simulink model "CruiseControlWithPID"  (R2021b)
settings: Solver=VariableStepAuto  StartTime=0.0  StopTime=50  FixedStep=0.01  RelTol=1e-3
PreLoadFcn:
  | clear;
  | CC_PID
values from neighbouring files (symbols this model uses):
  CC_b_Cn = 50    [CC_PID.m]
  CC_m_Cn = 1000    [CC_PID.m]
settings Model: Creator=banashreen  LastModifiedBy=Dell-pc
settings SolverCC: AlgebraicLoopSolver=TrustRegion
settings DataIOCC: ReturnWorkspaceOutputs=off
settings DebuggingCC: SFMachineParentedDataDiag=warning  ArithmeticOperatorsInVariantConditions=warning
settings SFSimCC: SimUseLocalCustomCode=off  CustomCodeUndefinedFunction=UseInterfaceOnly
settings RTWCC: RTWUseLocalCustomCode=off
settings ConfigComp: CovScope=ReferencedModels  CovIncludeTopModel=off

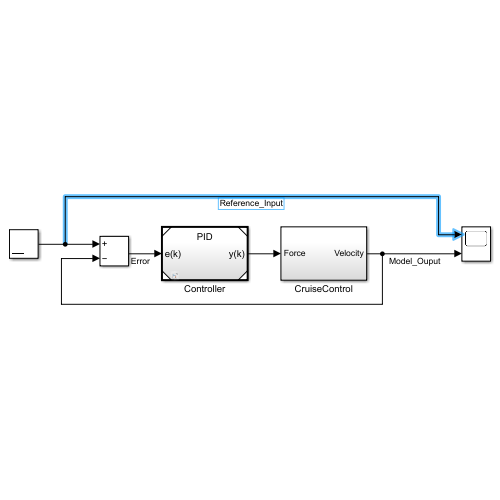
[thumbnail: Simulink's stored preview of the top-level diagram]
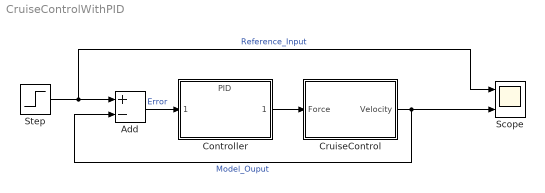
== system CruiseControlWithPID ==
  Add : Sum  Inputs=+-
  Controller : ModelReference  ModelNameDialog=PID.slx  SimulationMode=Normal  ShowModelTerminatePort=on  ModelReferenceVersion=9.3
  CruiseControl : Subsystem
  Scope : Scope  NumInputPorts=2
  Step : Step  Time=5  After=100  SampleTime=0
  wires:
  Step/1 -> Scope/1, Add/1  "Reference_Input"
  CruiseControl/1(Velocity) -> Add/2, Scope/2  "Model_Ouput"
  Controller/1 -> CruiseControl/1(Force)
  Add/1 -> Controller/1  "Error"

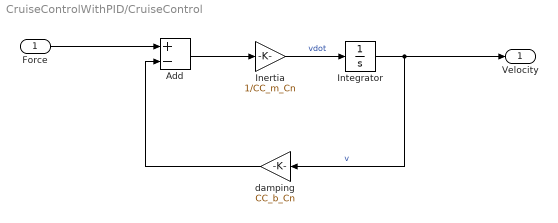
== system CruiseControlWithPID/CruiseControl ==
  Force : Inport
  Add : Sum  Inputs=+-
  Inertia : Gain  Gain=1/CC_m_Cn
  Integrator : Integrator
  damping : Gain  Gain=CC_b_Cn
  Velocity : Outport  VectorParamsAs1DForOutWhenUnconnected=off
  wires:
  Force/1 -> Add/1
  Add/1 -> Inertia/1
  Inertia/1 -> Integrator/1  "vdot"
  damping/1 -> Add/2
  Integrator/1 -> Velocity/1, damping/1  "v"
